simulink library "hydroInversionCoef_cl"  (R2022a)
settings: Solver=VariableStepAuto  StartTime=0.0  StopTime=10.0  RelTol=1e-3
undefined symbols (not defined in the file): vhcl
libraries: vrlib x2, vectorNormalizer_ul x2, matrix_library x1, alphaBetaLE_ul x1, localApparentWind_ul x1, rotateAboutVec x1, wakeEffect_ul x1
settings Model: Creator=adabney  LastModifiedBy=adabney

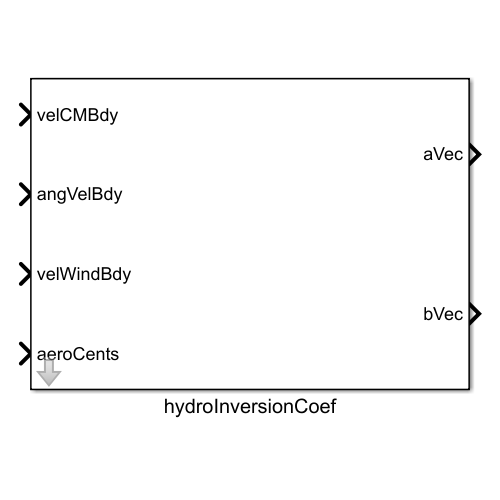
[thumbnail: Simulink's stored preview of the top-level diagram]
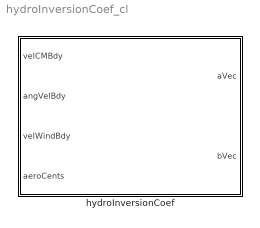
== system hydroInversionCoef_cl ==
  hydroInversionCoef : Subsystem  mask{aeroStruct=0}
      mask prompts: aeroStruct "Aero-surface"

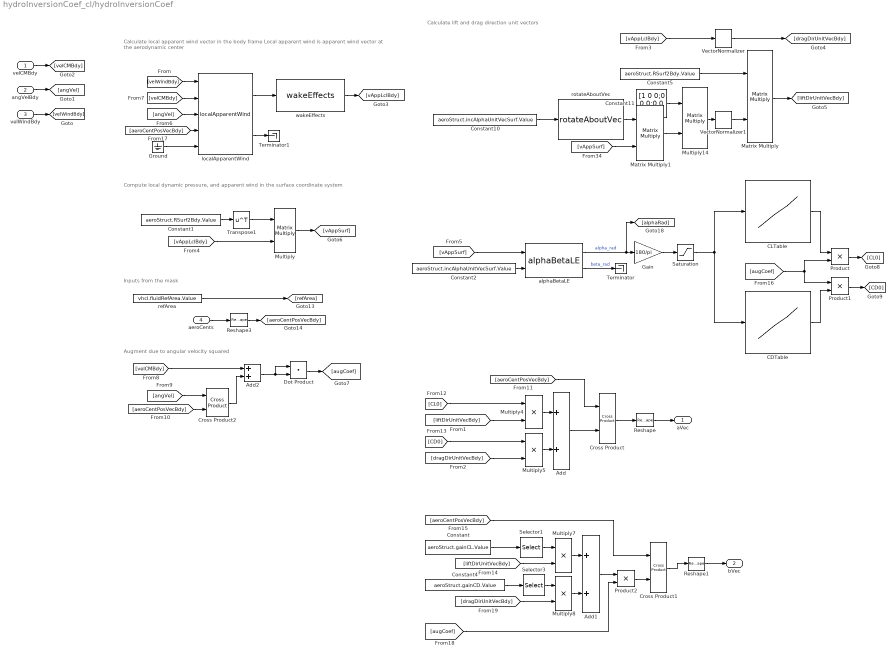
== system hydroInversionCoef_cl/hydroInversionCoef ==
  note: Inputs from the mask
  note: Calculate lift and drag direction unit vectors
  note: Augment due to angular velocity squared
  note: Calculate local apparent wind vector in the body frame
      | Local apparent wind is apparent wind vector at the aerodynamic center
  note: Compute local dynamic pressure,
      | and apparent wind in the surface coordinate system
  velCMBdy : Inport
  angVelBdy : Inport  Port=2
  velWindBdy : Inport  Port=3
  aeroCents : Inport  Port=4
  Add : Sum
  Add1 : Sum
  Add2 : Sum
  CDTable : Lookup_n-D  NumberOfTableDimensions=1  LookupTableObject=CLTable  BreakpointsForDimension1=aeroStruct.alpha.Value  Table=aeroStruct.CD.Value  ExtrapMethod=Clip  UseLastTableValue=on  InternalRulePriority=Speed  RndMeth=Simplest
  CLTable : Lookup_n-D  NumberOfTableDimensions=1  LookupTableObject=CLTable  BreakpointsForDimension1=aeroStruct.alpha.Value  Table=aeroStruct.CL.Value  ExtrapMethod=Clip  UseLastTableValue=on  InternalRulePriority=Speed  RndMeth=Simplest
  Constant : Constant  Value=aeroStruct.gainCL.Value
  Constant1 : Constant  Value=aeroStruct.RSurf2Bdy.Value
  Constant10 : Constant  Value=aeroStruct.incAlphaUnitVecSurf.Value
  Constant11 : Constant  Value=[1 0 0;0 0 0;0 0 1]
  Constant2 : Constant  Value=aeroStruct.incAlphaUnitVecSurf.Value
  Constant4 : Constant  Value=aeroStruct.gainCD.Value
  Constant5 : Constant  Value=aeroStruct.RSurf2Bdy.Value
  Cross Product : vrlib/Utilities/Cross Product
  Cross Product1 : vrlib/Utilities/Cross Product
  Cross Product2 : matrix_library/Cross Product
      settings: SourceProductBaseCode=SL
  Dot Product : DotProduct  OutDataTypeStr=Inherit: Inherit via internal rule
  Gain : Gain  Gain=180/pi
  Ground : Ground
  Matrix Multiply : Product  Multiplication=Matrix(*)
  Matrix Multiply1 : Product  Multiplication=Matrix(*)
  Multiply : Product  Multiplication=Matrix(*)
  Multiply14 : Product  Multiplication=Matrix(*)
  Multiply{4..5,7..8} (4 alike) : Product
  Product : Product
  Product1 : Product
  Product2 : Product
  Reshape : Reshape  OutputDimensionality=Column vector (2-D)
  Reshape1 : Reshape  OutputDimensionality=Column vector (2-D)
  Reshape3 : Reshape  OutputDimensionality=Column vector (2-D)
  Saturation : Saturate  UpperLimit=90  LowerLimit=-90
  Selector1 : Selector  InputPortWidth=3  IndexOptions=Index vector (dialog)  Indices=2  OutputSizes=1
  Selector3 : Selector  InputPortWidth=3  IndexOptions=Index vector (dialog)  Indices=2  OutputSizes=1
  Terminator : Terminator
  Terminator1 : Terminator
  Transpose1 : Math  Operator=transpose  SignedPower=on
  "VectorNormalizer " : vectorNormalizer_ul/VectorNormalizer   SystemSampleTime=-1  VariantActivationTime=update diagram  Latency=0  AutoFrameSizeCalculation=off
  VectorNormalizer1 : vectorNormalizer_ul/VectorNormalizer   SystemSampleTime=-1  VariantActivationTime=update diagram  Latency=0  AutoFrameSizeCalculation=off
  alphaBetaLE : alphaBetaLE_ul/alphaBetaLE  SystemSampleTime=-1  VariantActivationTime=update diagram  Latency=0  AutoFrameSizeCalculation=off
  localApparentWind : localApparentWind_ul/localApparentWind  SystemSampleTime=-1  VariantActivationTime=update diagram  Latency=0  AutoFrameSizeCalculation=off
  refArea : Constant  Value=vhcl.fluidRefArea.Value
  rotateAboutVec : rotateAboutVec/rotateAboutVec  ang=90
  wakeEffects : wakeEffect_ul/wakeEffects  SystemSampleTime=-1  VariantActivationTime=update diagram  Latency=0  AutoFrameSizeCalculation=off
  aVec : Outport  PortDimensions=[3 1]  VectorParamsAs1DForOutWhenUnconnected=off
  bVec : Outport  Port=2  PortDimensions=[3 1]  VectorParamsAs1DForOutWhenUnconnected=off
  wires:
  velCMBdy/1 -> [velCMBdy]
  angVelBdy/1 -> [angVel]
  Selector3/1 -> Multiply8/1
  [velWindBdy] -> localApparentWind/1
  Product2/1 -> Cross Product1/2
  CLTable/1 -> Product/1
  [augCoef] -> Product2/2
  Add1/1 -> Product2/1
  [velCMBdy] -> Add2/1
  Product1/1 -> [CD0]
  CDTable/1 -> Product1/2
  [liftDirUnitVecBdy] -> Multiply4/2
  Matrix Multiply/1 -> [liftDirUnitVecBdy]
  Multiply5/1 -> Add/2
  Add2/1 -> Dot Product/2, Dot Product/1
  [CD0] -> Multiply5/1
  [liftDirUnitVecBdy] -> Multiply7/2
  Selector1/1 -> Multiply7/1
  Matrix Multiply1/1 -> Multiply14/2
  Constant5/1 -> Matrix Multiply/1
  Reshape1/1 -> bVec/1
  "VectorNormalizer "/1 -> [dragDirUnitVecBdy]
  [CL0] -> Multiply4/1
  VectorNormalizer1/1 -> Matrix Multiply/2
  Constant1/1 -> Transpose1/1
  aeroCents/1 -> Reshape3/1
  Multiply/1 -> [vAppSurf]
  Constant2/1 -> alphaBetaLE/2
  [aeroCentPosVecBdy] -> Cross Product1/1
  Constant11/1 -> Multiply14/1
  [vAppSurf] -> Matrix Multiply1/2
  [dragDirUnitVecBdy] -> Multiply5/2
  Multiply14/1 -> VectorNormalizer1/1
  [aeroCentPosVecBdy] -> localApparentWind/4
  [velCMBdy] -> localApparentWind/2
  localApparentWind/2 -> Terminator1/1
  Multiply4/1 -> Add/1
  alphaBetaLE/1 -> Gain/1, [alphaRad]  "alpha_rad"
  Saturation/1 -> CLTable/1, CDTable/1
  Ground/1 -> localApparentWind/5
  alphaBetaLE/2 -> Terminator/1  "beta_rad"
  Multiply8/1 -> Add1/2
  Multiply7/1 -> Add1/1
  [vAppSurf] -> alphaBetaLE/1
  localApparentWind/1 -> wakeEffects/1
  Cross Product2/1 -> Add2/2
  Reshape/1 -> aVec/1
  Gain/1 -> Saturation/1
  wakeEffects/1 -> [vAppLclBdy]
  [dragDirUnitVecBdy] -> Multiply8/2
  Dot Product/1 -> [augCoef]
  Reshape3/1 -> [aeroCentPosVecBdy]
  [aeroCentPosVecBdy] -> Cross Product2/2
  [angVel] -> localApparentWind/3
  refArea/1 -> [refArea]
  [vAppLclBdy] -> Multiply/2
  Constant4/1 -> Selector3/1
  Transpose1/1 -> Multiply/1
  Cross Product/1 -> Reshape/1
  Add/1 -> Cross Product/2
  [augCoef] -> Product/2, Product1/1
  [angVel] -> Cross Product2/1
  Product/1 -> [CL0]
  rotateAboutVec/1 -> Matrix Multiply1/1
  Constant/1 -> Selector1/1
  [aeroCentPosVecBdy] -> Cross Product/1
  Constant10/1 -> rotateAboutVec/1
  velWindBdy/1 -> [velWindBdy]
  Cross Product1/1 -> Reshape1/1
  [vAppLclBdy] -> "VectorNormalizer "/1
